simulink model "DTMF"  (R2017b)
settings: Solver=VariableStepAuto  StartTime=0.0  StopTime=205  RelTol=1e-3
values from neighbouring files (symbols this model uses):
  A1 = cos(omega1)    [DualToneMultiFrequency.m]
  A2 = cos(omega2)    [DualToneMultiFrequency.m]
libraries: dspsrcs4 x2
settings Model: Creator=HP  LastModifiedBy=HP

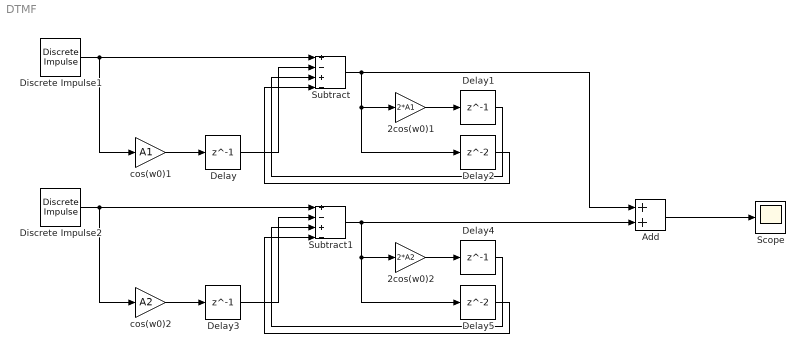
== system DTMF ==
  2cos(w0)1 : Gain  Gain=2*A1
  2cos(w0)2 : Gain  Gain=2*A2
  Add : Sum
  Delay{,1,3..4} (4 alike) : Delay  DelayLength=1
  Delay2 : Delay
  Delay5 : Delay
  Discrete Impulse1 : dspsrcs4/Discrete  Impulse  Delay=0  SampleTime=1  FrameSample=1  OutputFrames=off  dataType=double  isSigned=on  wordLen=16  udDataType=sfix(16)  fracBitsMode=Best precision  numFracBits=15  OutDataTypeStr=double  LastOutDataTypeStr=double
  Discrete Impulse2 : dspsrcs4/Discrete  Impulse  Delay=0  SampleTime=1  FrameSample=1  OutputFrames=off  dataType=double  isSigned=on  wordLen=16  udDataType=sfix(16)  fracBitsMode=Best precision  numFracBits=15  OutDataTypeStr=double  LastOutDataTypeStr=double
  Scope : Scope
  Subtract : Sum  Inputs=+-+-
  Subtract1 : Sum  Inputs=+-+-
  cos(w0)1 : Gain  Gain=A1
  cos(w0)2 : Gain  Gain=A2
  wires:
  cos(w0)1/1 -> Delay/1
  Discrete Impulse1/1 -> cos(w0)1/1, Subtract/1
  Delay/1 -> Subtract/2
  Subtract/1 -> Delay2/1, 2cos(w0)1/1, Add/1
  2cos(w0)1/1 -> Delay1/1
  Delay2/1 -> Subtract/4
  Delay1/1 -> Subtract/3
  Delay5/1 -> Subtract1/4
  Subtract1/1 -> Add/2, Delay5/1, 2cos(w0)2/1
  Delay3/1 -> Subtract1/2
  Delay4/1 -> Subtract1/3
  2cos(w0)2/1 -> Delay4/1
  Discrete Impulse2/1 -> cos(w0)2/1, Subtract1/1
  cos(w0)2/1 -> Delay3/1
  Add/1 -> Scope/1
